simulink model "przyklad_mateusz"  (R2023a)
settings: Solver=ode1  StartTime=0.0  StopTime=inf  FixedStep=0.0001  RelTol=1e-3  EnableMultiTasking=on
undefined symbols (not defined in the file): DiscIntNeverNeededParam, sigbuilder_block
libraries: stm32f4xxblockslib x8, simulink x7, stm32blockslib x6, stmutilitieslib x3, stm32f7xxblockslib x3
(part 1 of 2)
settings Model: STM32="{\"PWMOutput\":[{\"ID\":\"stm:582\"},{\"ID\":\"stm:3\"},{\"ID\":\"stm0x2810x29OLD:3\"},{\"ID\":\"stm0x2810x29OLD:582\"}],\"DigitalPortRead\":[{\"ID\":\"stm:1051\"},{\"ID\":\"stm:7\"},{\"ID\":\"stm:347\"},{\"ID\":\"stm0x2810x29:7\"},{\"ID\":\"stm0x2810x29OLD:1051\"},{\"ID\":\"stm0x2810x29OLD:7\"},{\"ID\":\"stm0x2810x29OLD:347\"}],\"DigitalPortWrite\":[{\"ID\":\"stm:1084\"},{\"ID\":\"stm:1\"},{\"ID\":\"stm:2\"},{\"ID\":\"stm:2305\"},{\"ID\":\"stm0x2810x29:2305\"},{\"ID\":\"stm0x2810x29OLD:2305\"},{\"ID\":\"stm0x2810x29OLD:1084\"},{\"ID\":\"stm0x2810x29OLD:1\"},{\"ID\":\"stm0x2810x29OLD:2\"}],\"EncoderBlock\":[{\"ID\":\"stm:382\"},{\"ID\":\"stm:667\"},{\"ID\":\"stm:421\"},{\"ID\":\"stm0x2810x29:667\"},{\"ID\":\"stm0x2810x29:421\"},{\"ID\":\"stm0x2810x29OLD:667\"},{\"ID\":\"stm0x2810x29OLD:421\"}],\"UARTWrite\":[{\"ID\":\"stm:1060\"},{\"ID\":\"stm:1095\"},{\"ID\":\"stm:1585\"},{\"ID\":\"stm0x2810x29:1095\"},{\"ID\":\"stm0x2810x29:1060\"},{\"ID\":\"stm0x2810x29OLD:1095\"},{\"ID\":\"stm0x2810x29OLD:1060\"},{\"ID\":\"stm0x2810x29OLD:1585\"}],\"UARTRead\":[{\"ID\":\"stm:1073\"},{\"ID\":\"stm0x2810x29OLD:1073\"}],\"HardwareInterrupt\":[{\"ID\":\"stm:216\"},{\"ID\":\"stm0x2810x29OLD:216\"}],\"AnalogInput\":[{\"ID\":\"stm:2303\"},{\"ID\":\"stm0x2810x29:2303\"},{\"ID\":\"stm0x2810x29OLD:2303\"}]}"  Creator=Susze  LastModifiedBy=matim
settings SolverCC: AutoInsertRateTranBlk=on
settings OptimizationCC: EnhancedBackFolding=on  PassReuseOutputArgsAs=Individual arguments  ZeroExternalMemoryAtStartup=off  ZeroInternalMemoryAtStartup=off  MaxStackSize=64  OptimizeBlockOrder=speed  DifferentSizesBufferReuse=on  OptimizationCustomize=off  EfficientTunableParamExpr=on
settings DebuggingCC: ParameterTunabilityLossMsg=error
settings HardwareCC: ProdBitPerPointer=32  ProdBitPerSizeT=32  ProdBitPerPtrDiffT=32  ProdLargestAtomicInteger=Long  ProdLargestAtomicFloat=Double  ProdWordSize=32  ProdLongLongMode=on  ProdHWDeviceType=ARM Compatible->ARM Cortex-M
settings SFSimCC: MATLABDynamicMemAlloc=off
settings RTWCC: Description=Embedded Coder  SystemTargetFile=ert.tlc  HardwareBoard=STM32F7xx Based (Double precision FPU)  TemplateMakefile=ert_default_tmf  Toolchain=GNU Tools for ARM Embedded Processors  GPUComputeCapability=5.0
settings CodeAppCC: ForceParamTrailComments=on  IgnoreCustomStorageClasses=off  OperatorAnnotations=on  SimulinkDataObjDesc=on  SFDataObjDesc=on  InsertBlockDesc=on
settings ERTTargetCC: TargetLangStandard=C99 (ISO)  CodeReplacementLibrary=ARM Cortex-M  SupportContinuousTime=on  SupportNonInlinedSFcns=on  ExtModeTransport=3  ExtModeStaticAlloc=on  ExtModeStaticAllocSize=2048  ExtModeMexFile=ext_xcp  ExtModeIntrfLevel=Level2 - Open

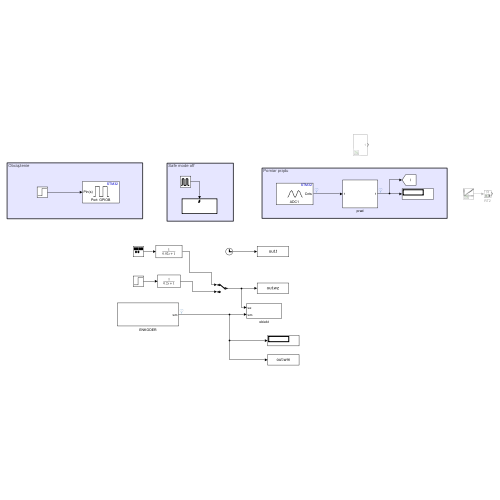
[thumbnail: Simulink's stored preview of the top-level diagram]
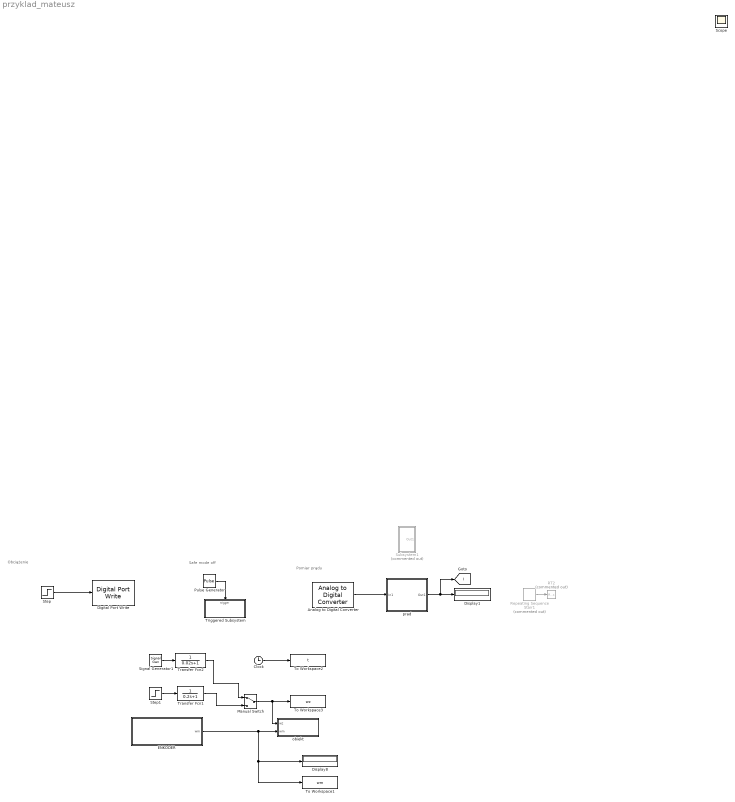
== system przyklad_mateusz ==
  note: Pomiar prądu
  note: Safe mode off
  note: Obciążenie
  Analog to Digital Converter : stm32f4xxblockslib/Analog to Digital Converter  ADCModule=ADC1  ConversionGroup=Regular  TriggerMode=Trigger and read  NumberOfConversions=1  EnableBufferConv=off  BufferLength=1  OutputStatus=off  SampleTime=-1  EnableSimPort=off  hoistedMaskSrc=ECSoC/ECSimCodegen/Analog to Digital Converter
      settings: LibrarySourceBlock=stm32f7xxblockslib/Analog to Digital Converter
  Clock : Clock
  Digital Port Write : stm32f4xxblockslib/Digital Port Write  PortName=GPIOB  PinNumber=[11]  ReadOperation=off  IOAsArray=on  EnableSimPort=off  hoistedMaskSrc=ECSoC/ECSimCodegen/Digital Port Write
      settings: LibrarySourceBlock=stm32f7xxblockslib/Digital Port Write
  Display1 : Display
  Display8 : Display
  ENKODER : Subsystem
  Manual Switch : ManualSwitch
  Pulse Generator : DiscretePulseGenerator  PulseType=Time based  Period=0.01  PulseWidth=10
  RT2 : RateTransition  Commented=on  OutPortSampleTime=0.0001
  Repeating Sequence Stair1 : simulink/Sources/Repeating Sequence Stair  Commented=on  OutValues=[0:0.1:1]  tsamp=5  OutMin=[]  OutMax=[]  OutDataTypeStr=double  OutputDataTypeScalingMode=double  OutDataType=fixdt(0,8)  ConRadixGroup=Best Precision: Vector-wise  OutScaling=2^-12
  Signal Generator1 : SignalGenerator  WaveForm=square  Amplitude=0  Frequency=0.5  Units=rad/sec
  Step : Step  Time=10  SampleTime=0
  Step1 : Step  After=0  SampleTime=0
  Subsystem1 : Subsystem  Commented=on
  To Workspace1 : ToWorkspace  VariableName=wm  SampleTime=-1
  To Workspace2 : ToWorkspace  VariableName=t  SampleTime=-1
  To Workspace3 : ToWorkspace  VariableName=wz  SampleTime=-1
  Transfer Fcn1 : TransferFcn  Denominator=[0.2 1]
  Transfer Fcn2 : TransferFcn  Denominator=[0.02 1]
  Triggered Subsystem : Subsystem  TreatAsAtomicUnit=on
  obiekt : Subsystem
  prad : Subsystem
  Scope : Scope
  tag scope: I=global
  wires:
  Pulse Generator/1 -> Triggered Subsystem/Trigger
  ENKODER/1(wm) -> Display8/1, To Workspace1/1, obiekt/2(wm)
  Clock/1 -> To Workspace2/1
  Manual Switch/1 -> obiekt/1(wz), To Workspace3/1
  Signal Generator1/1 -> Transfer Fcn2/1
  Transfer Fcn2/1 -> Manual Switch/1
  Step1/1 -> Transfer Fcn1/1
  Transfer Fcn1/1 -> Manual Switch/2
  Repeating Sequence Stair1/1 -> RT2/1
  Analog to Digital Converter/1 -> prad/1(In1)
  prad/1(Out1) -> [I], Display1/1
  Step/1 -> Digital Port Write/1

== system przyklad_mateusz/ENKODER ==
  Constant : Constant  Value=65536
  Constant1 : Constant  Value=1250
  Detect Rise Positive : simulink/Logic and Bit Operations/Detect Rise Positive  vinit=0  OutDataTypeStr=boolean
  Divide : Product  Inputs=*/
  Encoder1 : stm32blockslib/Encoder  TimerModule=TIM4  EnableResetInput=on  OutputDirection=on  SampleTime=-1
      settings: LibrarySourceBlock=stm32f7xxblockslib/Encoder
  Minus : Sum  Inputs=+-
  Pulse Generator : DiscretePulseGenerator  PulseType=Time based  Period=0.01  PulseWidth=10
  Switch : Switch  Criteria=u2 > Threshold  SaturateOnIntegerOverflow=off  InputSameDT=off
  Triggered Subsystem : Subsystem  TreatAsAtomicUnit=on
  Unit Delay : UnitDelay  SampleTime=-1  HasFrameUpgradeWarning=on
  wm : Outport
  wires:
  Detect Rise Positive/1 -> Unit Delay/1
  Switch/1 -> Triggered Subsystem/1(In1)
  Encoder1/2 -> Switch/2
  Encoder1/1 -> Switch/3, Minus/1
  Constant/1 -> Minus/2
  Minus/1 -> Switch/1
  Constant1/1 -> Divide/2
  Triggered Subsystem/1(wm) -> Divide/1
  Pulse Generator/1 -> Detect Rise Positive/1, Triggered Subsystem/Trigger
  Unit Delay/1 -> Encoder1/1
  Divide/1 -> wm/1

== system przyklad_mateusz/Subsystem1 ==
  Byte Pack1 : stmutilitieslib/Byte Pack  Commented=on  datatypes={'uint8';'uint8';'uint8';'uint8';'uint8'}  byteAlign=1  blockPlatform=stm32f4discovery
  Constant5 : Constant  Commented=on  Value=170  OutDataTypeStr=uint8
  Constant6 : Constant  Commented=on  Value=12  OutDataTypeStr=uint8
  Constant7 : Constant  Commented=on  Value=5  OutDataTypeStr=uint8
  Constant8 : Constant  Commented=on  Value=0  OutDataTypeStr=uint8
  Constant9 : Constant  Commented=on  Value=0  OutDataTypeStr=uint8
  RT : RateTransition  Commented=on  OutPortSampleTime=0.0001
  Repeating Sequence Stair : simulink/Sources/Repeating Sequence Stair  Commented=on  OutValues=[0:0.1:1]  tsamp=5  OutMin=[]  OutMax=[]  OutDataTypeStr=double  OutputDataTypeScalingMode=double  OutDataType=fixdt(0,8)  ConRadixGroup=Best Precision: Vector-wise  OutScaling=2^-12
  Signal Builder2 : Subsystem  Tag=STV Subsys  Commented=on  LoadFcn=sigbuilder_block('load');  StartFcn=sigbuilder_block('start');  StopFcn=sigbuilder_block('stop');  ClipboardFcn=sigbuilder_block('clipboard');  mask(Sigbuilder block){tuvar=[0:10]}
      mask help: Simulink:masks:SigbuilderBlock_MD
      mask init:
      | if ~strcmp(get_param(bdroot(gcbh),'SimulationStatus'),'stopped') tuvar = sigbuilder_block('maskInit'); end
      settings: CopyFcn=sigbuilder_block('copy');  DeleteFcn=sigbuilder_block('delete');  ModelCloseFcn=sigbuilder_block('modelClose');  PreSaveFcn=sigbuilder_block('preSave');  PauseFcn=sigbuilder_block('pause');  ContinueFcn=sigbuilder_block('continue');  NameChangeFcn=sigbuilder_block('namechange');  OpenFcn=sigbuilder_block('open',[5.4 36 1141.2 516.6 ]);  CloseFcn=sigbuilder_block('close');
      mask Display: plot(0, 0, 100, 100,[2, 2, 32, 32, 2], [68, 8, 8, 68, 68],[32, 2], [38, 38], [32, 19, 2],[53, 60, 44], [32, 17, 17, 2],[16, 16, 31, 31]);txt = getActiveGroup(gcbh);text(2, 100, txt,'verticalAlignment', 'top');
  Step3 : Step  Commented=on  Time=0.01  SampleTime=0
  Subsystem : Subsystem  Commented=on
  UART/USART Write1 : stm32blockslib/UART//USART Write  Commented=on  UARTModule=UART4  LengthOfDataToSend=off  BlockingMode=off  BlockingTimeout=0.1  OutputStatus=off
      settings: LibrarySourceBlock=stm32f7xxblockslib/UART//USART Write
  Out1 : Outport
  wires:
  Constant8/1 -> Byte Pack1/4
  RT/1 -> Out1/1
  Constant9/1 -> Byte Pack1/5  "prędkość 0-100"
  Constant5/1 -> Byte Pack1/1
  Constant6/1 -> Byte Pack1/2
  Byte Pack1/1 -> UART/USART Write1/1
  Repeating Sequence Stair/1 -> RT/1
  Constant7/1 -> Byte Pack1/3

== system przyklad_mateusz/Triggered Subsystem ==
  Trigger : TriggerPort  VariantControl=(inherit)
  Byte Pack1 : stmutilitieslib/Byte Pack  datatypes={'uint8';'uint8';'uint8'}  byteAlign=1  blockPlatform=stm32f4discovery
  Constant7 : Constant  Value=170  OutDataTypeStr=uint8
  Constant8 : Constant  Value=12  OutDataTypeStr=uint8
  Constant9 : Constant  Value=3  OutDataTypeStr=uint8
  UART/USART Write1 : stm32blockslib/UART//USART Write  UARTModule=UART4  LengthOfDataToSend=off  BlockingMode=off  BlockingTimeout=0.1  OutputStatus=off
      settings: LibrarySourceBlock=stm32f7xxblockslib/UART//USART Write
  wires:
  Constant9/1 -> Byte Pack1/3
  Constant8/1 -> Byte Pack1/2
  Byte Pack1/1 -> UART/USART Write1/1
  Constant7/1 -> Byte Pack1/1

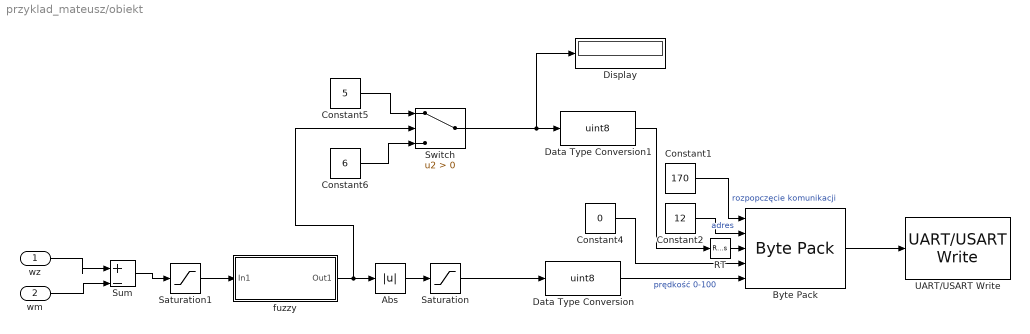
== system przyklad_mateusz/obiekt ==
  wz : Inport
  wm : Inport  Port=2
  Abs : Abs  SaturateOnIntegerOverflow=off
  Byte Pack : stmutilitieslib/Byte Pack  datatypes={'uint8';'uint8';'uint8';'uint8';'uint8'}  byteAlign=1  blockPlatform=stm32f4discovery
  Constant1 : Constant  Value=170  OutDataTypeStr=uint8
  Constant2 : Constant  Value=12  OutDataTypeStr=uint8
  Constant4 : Constant  Value=0  OutDataTypeStr=uint8
  Constant5 : Constant  Value=5  OutDataTypeStr=uint8
  Constant6 : Constant  Value=6  OutDataTypeStr=uint8
  Data Type Conversion : DataTypeConversion  OutDataTypeStr=uint8  SaturateOnIntegerOverflow=off  RndMeth=Floor
  Data Type Conversion1 : DataTypeConversion  OutDataTypeStr=uint8  SaturateOnIntegerOverflow=off  RndMeth=Floor
  Display : Display
  RT : RateTransition  OutPortSampleTime=0.0001
  Saturation : Saturate  UpperLimit=100  LowerLimit=0
  Saturation1 : Saturate  UpperLimit=1  LowerLimit=-1
  Sum : Sum  Inputs=|+-
  Switch : Switch  Criteria=u2 > Threshold  SaturateOnIntegerOverflow=off  InputSameDT=off
  UART/USART Write : stm32blockslib/UART//USART Write  UARTModule=UART4  LengthOfDataToSend=off  BlockingMode=off  BlockingTimeout=0.1  OutputStatus=off
      settings: LibrarySourceBlock=stm32f7xxblockslib/UART//USART Write
  fuzzy : Subsystem
  wires:
  Sum/1 -> Saturation1/1
  wz/1 -> Sum/1
  wm/1 -> Sum/2
  Constant2/1 -> Byte Pack/2  "adres"
  Constant1/1 -> Byte Pack/1  "rozpopczęcie komunikacji"
  Byte Pack/1 -> UART/USART Write/1
  Constant4/1 -> Byte Pack/4
  Data Type Conversion/1 -> Byte Pack/5  "prędkość 0-100"
  Constant5/1 -> Switch/1
  Constant6/1 -> Switch/3
  Switch/1 -> Data Type Conversion1/1, Display/1
  Data Type Conversion1/1 -> RT/1
  RT/1 -> Byte Pack/3
  Abs/1 -> Saturation/1
  Saturation1/1 -> fuzzy/1(In1)
  fuzzy/1(Out1) -> Abs/1, Switch/2
  Saturation/1 -> Data Type Conversion/1

== system przyklad_mateusz/prad ==
  In1 : Inport
  Constant : Constant  Value=1.65
  Gain : Gain  Gain=0.00080586
  Gain1 : Gain  Gain=15.15
  Sum : Sum  Inputs=|+-
  Transfer Fcn3 : TransferFcn  Denominator=[0.2 1]
  Out1 : Outport
  wires:
  In1/1 -> Gain/1
  Gain/1 -> Sum/1
  Constant/1 -> Sum/2
  Sum/1 -> Gain1/1
  Gain1/1 -> Transfer Fcn3/1
  Transfer Fcn3/1 -> Out1/1

== system przyklad_mateusz/ENKODER/Triggered Subsystem ==
  In1 : Inport
  Trigger : TriggerPort  VariantControl=(inherit)
  Gain : Gain  Gain=3
  wm : Outport
  wires:
  In1/1 -> Gain/1
  Gain/1 -> wm/1

== system przyklad_mateusz/Subsystem1/Signal Builder2 ==
  Demux : Demux  Tag=STV Demux  Outputs=1
      settings: DisplayOption=none
  FromWs : FromWorkspace  Tag=STV FromWs  VariableName=tuvar
      SigBuilderData=|
      | common.afterFinalStr = 'Extrapolate'
      | common.sampleTime = 0
      | dataSet.timeRange = [0 60]
      | dataSet.name = 'Group 1'
      | sbobj.Groups.Name = 'Group 1'
      | sbobj.Groups.Signals.Name = 'Prędkość'
      | sbobj.Groups.Signals.XData = [0 2 2 8 8 14 14 20 20 26 26 32 32 38 38 55.75 55.75 60]
      | sbobj.Groups.Signals.YData = [0 0 0.4 0.4 -0.395 -0.395 0.405 0.405 -0.4 -0.4 0.4 0.4 -0.4 -0.4 0.4 0.4 0 0]
      | sbobj.Groups.TimeRange = [0 60]
  Prędkość : Outport  Tag=STV Outport
  wires:
  Demux/1 -> Prędkość/1
  FromWs/1 -> Demux/1

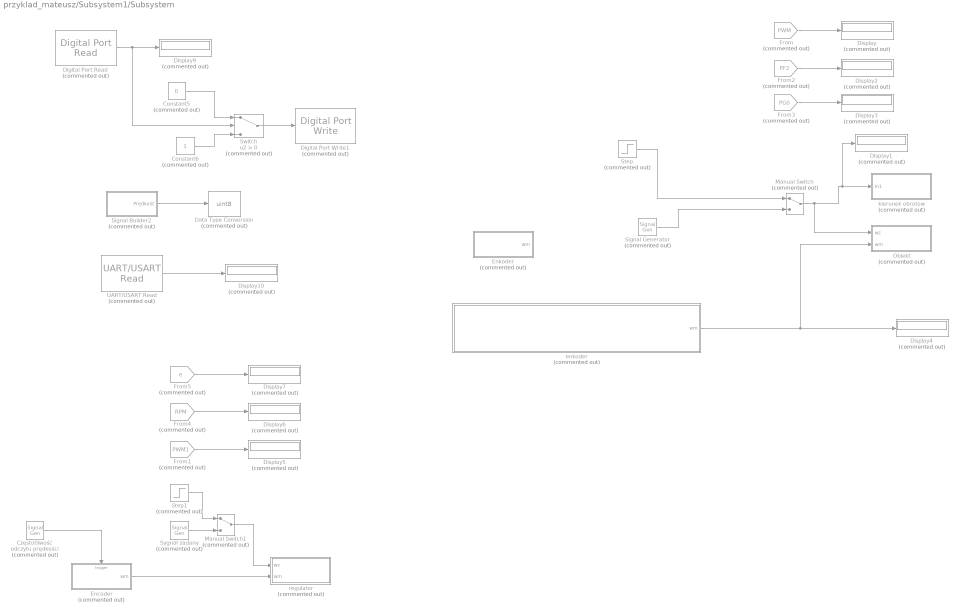
== system przyklad_mateusz/Subsystem1/Subsystem ==
  Constant5 : Constant  Commented=on  Value=0
  Constant6 : Constant  Commented=on
  Częstotliwość odczytu prędkości : SignalGenerator  Commented=on  WaveForm=square  Frequency=100
  Data Type Conversion : DataTypeConversion  Commented=on  OutDataTypeStr=uint8  SaturateOnIntegerOverflow=off  RndMeth=Floor
  Digital Port Read : stm32f4xxblockslib/Digital Port Read  Commented=on  PortName=GPIOB  PinNumber=[9]  ReadOperation=on  IOAsArray=on  SampleTime=-1  EnableSimPort=off  hoistedMaskSrc=ECSoC/ECSimCodegen/Digital Port Read
      settings: LibrarySourceBlock=stm32f7xxblockslib/Digital Port Read
  Digital Port Write1 : stm32f4xxblockslib/Digital Port Write  Commented=on  PortName=GPIOB  PinNumber=[8]  ReadOperation=off  IOAsArray=on  EnableSimPort=off  hoistedMaskSrc=ECSoC/ECSimCodegen/Digital Port Write
      settings: LibrarySourceBlock=stm32f7xxblockslib/Digital Port Write
  Display{,1..7,9..10} (10 alike) : Display  Commented=on
  Encoder : Subsystem  Commented=on  TreatAsAtomicUnit=on
  Enkoder : Subsystem  Commented=on
  From : From  Commented=on  GotoTag=PWM  TagVisibility=global
  From1 : From  Commented=on  GotoTag=PWM1
  From2 : From  Commented=on  GotoTag=PF2  TagVisibility=global
  From3 : From  Commented=on  GotoTag=PG0  TagVisibility=global
  From4 : From  Commented=on  GotoTag=RPM  TagVisibility=global
  From5 : From  Commented=on  GotoTag=e
  Manual Switch : ManualSwitch  Commented=on
  Manual Switch1 : ManualSwitch  Commented=on
  Obiekt : Subsystem  Commented=on
  Signal Generator : SignalGenerator  Commented=on  WaveForm=square  Frequency=0.1  Units=rad/sec
  Signal Builder2 : Subsystem  Tag=STV Subsys  Commented=on  LoadFcn=sigbuilder_block('load');  StartFcn=sigbuilder_block('start');  StopFcn=sigbuilder_block('stop');  ClipboardFcn=sigbuilder_block('clipboard');  mask(Sigbuilder block){tuvar=[0:10]}
      mask help: Simulink:masks:SigbuilderBlock_MD
      mask init:
      | if ~strcmp(get_param(bdroot(gcbh),'SimulationStatus'),'stopped') tuvar = sigbuilder_block('maskInit'); end
      settings: CopyFcn=sigbuilder_block('copy');  DeleteFcn=sigbuilder_block('delete');  ModelCloseFcn=sigbuilder_block('modelClose');  PreSaveFcn=sigbuilder_block('preSave');  PauseFcn=sigbuilder_block('pause');  ContinueFcn=sigbuilder_block('continue');  NameChangeFcn=sigbuilder_block('namechange');  OpenFcn=sigbuilder_block('open',[0 36 1152 555.6 ]);  CloseFcn=sigbuilder_block('close');
      mask Display: plot(0, 0, 100, 100,[2, 2, 32, 32, 2], [68, 8, 8, 68, 68],[32, 2], [38, 38], [32, 19, 2],[53, 60, 44], [32, 17, 17, 2],[16, 16, 31, 31]);txt = getActiveGroup(gcbh);text(2, 100, txt,'verticalAlignment', 'top');
  Step : Step  Commented=on  SampleTime=0
  Step1 : Step  Commented=on  After=200  SampleTime=0
  Switch : Switch  Commented=on  Criteria=u2 > Threshold  SaturateOnIntegerOverflow=off  InputSameDT=off
  Sygnał zadany : SignalGenerator  Commented=on  WaveForm=square  Amplitude=0.5  Frequency=0.1
  UART/USART Read : stm32blockslib/UART//USART Read  Commented=on  UARTModule=UART4  DataType=uint8  DataLength=1  BlockingMode=off  BlockingTimeout=0.1  OutputLength=off  OutputStatus=off  SampleTime=-1
      settings: LibrarySourceBlock=stm32f7xxblockslib/UART//USART Read
  enkoder : Subsystem  Commented=on
  kierunek obrotow : Subsystem  Commented=on
  regulator : Subsystem  Commented=on
  wires:
  Digital Port Read/1 -> Switch/2, Display9/1
  Switch/1 -> Digital Port Write1/1
  Constant5/1 -> Switch/1
  Signal Builder2/1(Prędkość) -> Data Type Conversion/1
  Constant6/1 -> Switch/3
  UART/USART Read/1 -> Display10/1
  Step1/1 -> Manual Switch1/1
  From5/1 -> Display7/1
  Częstotliwość odczytu prędkości/1 -> Encoder/Trigger
  Sygnał zadany/1 -> Manual Switch1/2
  Manual Switch1/1 -> regulator/1(wz)
  From1/1 -> Display5/1
  Encoder/1(wm) -> regulator/2(wm)
  From4/1 -> Display6/1
  From2/1 -> Display2/1
  From3/1 -> Display3/1
  enkoder/1(wm) -> Obiekt/2(wm), Display4/1
  Step/1 -> Manual Switch/1
  Signal Generator/1 -> Manual Switch/2
  Manual Switch/1 -> Obiekt/1(wz), Display1/1, kierunek obrotow/1(In1)
  From/1 -> Display/1

== system przyklad_mateusz/obiekt/fuzzy ==
  In1 : Inport
  Discrete Derivative : simulink/Discrete/Discrete Derivative  gainval=1.0  ICPrevScaledInput=0.0  OutMin=[]  OutMax=[]  OutDataType=fixdt(1, 16)  OutScaling=2^-10  DoSatur=off
  Discrete-Time Integrator : DiscreteIntegrator  SampleTime=-1  ICPrevOutput=DiscIntNeverNeededParam  ICPrevScaledInput=DiscIntNeverNeededParam
  Fuzzy Logic Controller : Subsystem  Commented=on
      mask help: Simulink:masks:GenSFuncDesc_MD
      mask Help: eval('feval(''rtwprivate'',''rtwhelpview'',''rtw_sfcn_block'')');
      mask Display:
      | iconStr = fuzzy.internal.utility.getMaskDisplayString;
      | eval(iconStr)
  Fuzzy Type 1 : Subsystem  Commented=on
  Fuzzy Type 2 : Subsystem
  Gain : Gain  Gain=2
  Gain1 : Gain  Gain=0.05
  Gain2 : Gain  Gain=300
  Mux : Mux  Commented=on  Inputs=2
  Saturation : Saturate  UpperLimit=1  LowerLimit=-1
  Saturation1 : Saturate  UpperLimit=1  LowerLimit=-1
  Out1 : Outport
  wires:
  In1/1 -> Discrete Derivative/1, Gain/1
  Gain/1 -> Saturation/1
  Discrete Derivative/1 -> Gain1/1
  Gain1/1 -> Saturation1/1
  Gain2/1 -> Discrete-Time Integrator/1
  Discrete-Time Integrator/1 -> Out1/1
  Mux/1 -> Fuzzy Logic Controller/1(in)
  Saturation1/1 -> Fuzzy Type 2/2(de1)
  Saturation/1 -> Fuzzy Type 2/1(e2)
  Fuzzy Type 2/1(du) -> Gain2/1

== system przyklad_mateusz/Subsystem1/Subsystem/Encoder ==
  Trigger : TriggerPort  TriggerType=falling  VariantControl=(inherit)
  Add : Sum
  Constant3 : Constant  Value=65536
  Display : Display
  Encoder : stm32blockslib/Encoder  TimerModule=TIM4  EnableResetInput=on  OutputDirection=on  SampleTime=-1
      settings: LibrarySourceBlock=stm32f7xxblockslib/Encoder
  Gain : Gain  Gain=6
  Subtract : Sum  Inputs=+-
  Subtract1 : Sum  Inputs=+-
  Switch : Switch  Criteria=u2 > Threshold  SaturateOnIntegerOverflow=off  InputSameDT=off
  Unit Delay : UnitDelay  SampleTime=-1  HasFrameUpgradeWarning=on
  wm : Outport
  tag scope: RPM=global
  wires:
  Subtract/1 -> Switch/2, Switch/1
  Switch/1 -> Gain/1
  Add/1 -> Switch/3
  Constant3/1 -> Subtract1/1
  Subtract1/1 -> Add/2
  Encoder/1 -> Unit Delay/1, Add/1, Subtract/1
  Unit Delay/1 -> Subtract1/2, Subtract/2
  Gain/1 -> [RPM], wm/1
  Encoder/2 -> Display/1

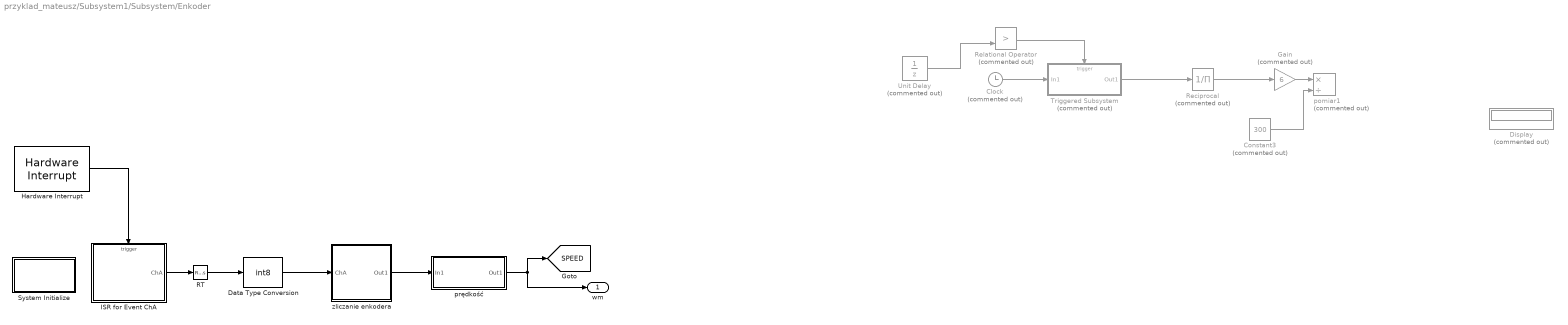
== system przyklad_mateusz/Subsystem1/Subsystem/Enkoder ==
  Clock : Clock  Commented=on
  Constant3 : Constant  Commented=on  Value=300
  Data Type Conversion : DataTypeConversion  OutDataTypeStr=int8  SaturateOnIntegerOverflow=off  RndMeth=Floor
  Display : Display  Commented=on
  Gain : Gain  Commented=on  Gain=6
  Hardware Interrupt : stm32f7xxblockslib/Hardware Interrupt  ISRGroup=External interrupts (EXTI)  ISRName=EXTI3_IRQHandler  ISRNumber=24  EventsList={ 'on', 'EXTI3 Event', '1'; 'off', 'Custom event', '2' }  SelectedEvents={'EXTI3 Event'}  TaskPriority=30  DisablePreemption=off  ClearInterruptFlagsAtEndOfEvent=off  InterruptDefinitionFile=$(TARGET_ROOT)/registry/interrupts/STM32F4xxBased_interrupts.xml  HardwareBoard=STM32F7xx Based  EnableSimPort=off
  ISR for Event ChA : Subsystem  TreatAsAtomicUnit=on
  RT : RateTransition  Deterministic=off  OutPortSampleTime=0.001
  Reciprocal : Product  Commented=on  Inputs=/
  Relational Operator : RelationalOperator  Commented=on  Operator=>  OutDataTypeStr=boolean  RndMeth=Simplest  InputSameDT=off
  System Initialize : Subsystem  mask(System Initialize){ShowInLibBrowser=0}
      mask prompts: ShowInLibBrowser "Simulink:masks:CustCodeMaskParam1_MP"
      settings: CopyFcn=cccopyfcn(gcb)  OpenFcn=ccopenfcn('System Initialize Function')
      mask Help: eval('feval(''rtwprivate'',''rtwhelpview'',''rtw_sys_initialize_block'')');
      mask Display: disp('System\nInitialize');
  Triggered Subsystem : Subsystem  Commented=on  TreatAsAtomicUnit=on
  Unit Delay : UnitDelay  Commented=on  SampleTime=-1  HasFrameUpgradeWarning=on
  pomiar1 : Product  Commented=on  Inputs=*/
  prędkość : Subsystem
  zliczanie enkodera : Subsystem
  wm : Outport
  tag scope: SPEED=global
  wires:
  Hardware Interrupt/1 -> ISR for Event ChA/Trigger
  Triggered Subsystem/1(Out1) -> Reciprocal/1
  Relational Operator/1 -> Triggered Subsystem/Trigger
  Clock/1 -> Triggered Subsystem/1(In1)
  Constant3/1 -> pomiar1/2
  Reciprocal/1 -> Gain/1
  Gain/1 -> pomiar1/1
  ? -> Relational Operator/1, Unit Delay/1
  Unit Delay/1 -> Relational Operator/2
  RT/1 -> Data Type Conversion/1
  Data Type Conversion/1 -> zliczanie enkodera/1(ChA)
  zliczanie enkodera/1(Out1) -> prędkość/1(In1)
  prędkość/1(Out1) -> wm/1, [SPEED]
  ISR for Event ChA/1(ChA) -> RT/1

== system przyklad_mateusz/Subsystem1/Subsystem/Obiekt ==
  wz : Inport
  wm : Inport  Port=2
  Constant : Constant  Value=80
  Manual Switch : ManualSwitch  CurrentSetting=0
  Moj : Subsystem
  PWM Output : stm32f7xxblockslib/PWM Output  TimerModule=TIM1  DutycycleUnits=Percentage  EnableChannel1=on  EnableChannel2=off  EnableChannel3=off  EnableChannel4=off  EnableChannel5=off  EnableChannel6=off  EnableCounterInput=off  EnableMainOutputInput=off  EnableFrequencyInput=off  SetRCAfterCE=off  OutputDirection=off  OutputMainOutputEnableStatus=off  SampleTime=0.1  EnableSimPort=off  EnableUpdateEvent=off  EnableCaptureCompare1Event=off  EnableCaptureCompare2Event=off  EnableCaptureCompare3Event=off  EnableCaptureCompare4Event=off  EnableTriggerEvent=off  EnableBreakEvent=off  EnableBreakEvent2=off  ProcessorFamily=STM32F7  hoistedMaskSrc=ECSoC/ECSimCodegen/PWM Output
  Saturation : Saturate  UpperLimit=100  LowerLimit=0
  Sum : Sum  Inputs=|+-
  tag scope: PWM=global
  wires:
  Sum/1 -> Moj/1(In1)
  Moj/1(Out1) -> Saturation/1
  wz/1 -> Sum/1
  wm/1 -> Sum/2
  Saturation/1 -> Manual Switch/2
  Constant/1 -> Manual Switch/1
  Manual Switch/1 -> [PWM], PWM Output/1

== system przyklad_mateusz/Subsystem1/Subsystem/Signal Builder2 ==
  Demux : Demux  Tag=STV Demux  Outputs=1
      settings: DisplayOption=none
  FromWs : FromWorkspace  Tag=STV FromWs  VariableName=tuvar
      SigBuilderData=|
      | common.afterFinalStr = 'Extrapolate'
      | common.sampleTime = 0
      | dataSet.timeRange = [0 40]
      | dataSet.name = 'Group 1'
      | sbobj.Groups.Name = 'Group 1'
      | sbobj.Groups.Signals.Name = 'Prędkość'
      | sbobj.Groups.Signals.XData = [0 5 5 10 10 15 15 20 20 25 25 30 30 35 35 40]
      | sbobj.Groups.Signals.YData = [0 0 20 20 30 30 40 40 50 50 60 60 70 70 80.2 80.2]
      | sbobj.Groups.TimeRange = [0 40]
  Prędkość : Outport  Tag=STV Outport
  wires:
  Demux/1 -> Prędkość/1
  FromWs/1 -> Demux/1

== system przyklad_mateusz/Subsystem1/Subsystem/enkoder ==
  Clock : Clock
  Constant3 : Constant  Value=300
  Data Type Conversion : DataTypeConversion  OutDataTypeStr=uint8  SaturateOnIntegerOverflow=off  RndMeth=Floor
  Digital Port Read : stm32f4xxblockslib/Digital Port Read  PortName=GPIOA  PinNumber=[3]  ReadOperation=on  IOAsArray=on  SampleTime=-1  EnableSimPort=off  hoistedMaskSrc=ECSoC/ECSimCodegen/Digital Port Read
      settings: LibrarySourceBlock=stm32f7xxblockslib/Digital Port Read
  Gain : Gain  Gain=6
  Reciprocal : Product  Inputs=/
  Relational Operator : RelationalOperator  Operator=>  OutDataTypeStr=boolean  RndMeth=Simplest  InputSameDT=off
  Triggered Subsystem : Subsystem  TreatAsAtomicUnit=on
  Unit Delay : UnitDelay  SampleTime=-1  HasFrameUpgradeWarning=on
  pomiar1 : Product  Inputs=*/
  wm : Outport
  wires:
  Digital Port Read/1 -> Relational Operator/1, Unit Delay/1
  Clock/1 -> Triggered Subsystem/1(In1)
  Triggered Subsystem/1(Out1) -> Reciprocal/1
  Unit Delay/1 -> Relational Operator/2
  Gain/1 -> pomiar1/1
  Reciprocal/1 -> Gain/1
  Constant3/1 -> pomiar1/2
  Relational Operator/1 -> Triggered Subsystem/Trigger
  pomiar1/1 -> wm/1

== system przyklad_mateusz/Subsystem1/Subsystem/kierunek obrotow ==
  In1 : Inport
  Digital Port Write : stm32f4xxblockslib/Digital Port Write  PortName=GPIOG  PinNumber=[0]  ReadOperation=off  IOAsArray=on  EnableSimPort=off  hoistedMaskSrc=ECSoC/ECSimCodegen/Digital Port Write
      settings: LibrarySourceBlock=stm32f7xxblockslib/Digital Port Write
  Digital Port Write1 : stm32f4xxblockslib/Digital Port Write  PortName=GPIOF  PinNumber=[2]  ReadOperation=off  IOAsArray=on  EnableSimPort=off  hoistedMaskSrc=ECSoC/ECSimCodegen/Digital Port Write
      settings: LibrarySourceBlock=stm32f7xxblockslib/Digital Port Write
  kierunek obrotów : Subsystem
  tag scope: PF2=global, PG0=global
  wires:
  In1/1 -> kierunek obrotów/1(u)
  kierunek obrotów/1(y) -> Digital Port Write/1, [PG0]
  kierunek obrotów/2(Out2) -> [PF2], Digital Port Write1/1

== system przyklad_mateusz/Subsystem1/Subsystem/regulator ==
  wz : Inport
  wm : Inport  Port=2
  Constant : Constant  Value=80
  Manual Switch : ManualSwitch  CurrentSetting=0
  PWM Output : stm32f7xxblockslib/PWM Output  TimerModule=TIM1  DutycycleUnits=Percentage  EnableChannel1=on  EnableChannel2=off  EnableChannel3=off  EnableChannel4=off  EnableChannel5=off  EnableChannel6=off  EnableCounterInput=off  EnableMainOutputInput=off  EnableFrequencyInput=off  SetRCAfterCE=off  OutputDirection=off  OutputMainOutputEnableStatus=off  SampleTime=0.1  EnableSimPort=off  EnableUpdateEvent=off  EnableCaptureCompare1Event=off  EnableCaptureCompare2Event=off  EnableCaptureCompare3Event=off  EnableCaptureCompare4Event=off  EnableTriggerEvent=off  EnableBreakEvent=off  EnableBreakEvent2=off  ProcessorFamily=STM32F7  hoistedMaskSrc=ECSoC/ECSimCodegen/PWM Output
  Saturation : Saturate  UpperLimit=100  LowerLimit=0
  Sum : Sum  Inputs=|+-
  fuzzy : Subsystem
  tag scope: PWM1=global, e=global
  wires:
  Sum/1 -> [e], fuzzy/1(In1)
  fuzzy/1(Out1) -> Saturation/1
  wz/1 -> Sum/1
  wm/1 -> Sum/2
  Saturation/1 -> Manual Switch/2
  Constant/1 -> Manual Switch/1
  Manual Switch/1 -> [PWM1], PWM Output/1

== system przyklad_mateusz/obiekt/fuzzy/Fuzzy Logic Controller ==
  in : Inport
  Fuzzy Logic Controller_sfcn : S-Function  FunctionName=Fuzzy0_sf  SFunctionModules=""  SFunctionDeploymentMode=off  EnableBusSupport=off  mask{rtw_sf_name=Fuzzy0_sf, showVar=off}
      mask prompts: rtw_sf_name "Simulink:masks:GenSFuncName_MP"; showVar "Simulink:masks:GenSFuncShowModuleList_MP"
      mask help: Simulink:masks:GenSFuncDesc_MD
      mask init:
      | displist = '';
      | if ~strcmp(get_param(gcb, 'FunctionName'), rtw_sf_name);
      |   set_param(gcb, 'FunctionName', rtw_sf_name);
      | end
      | % Check if we are generating code
      | rtw_mode = false;
      | if strcmpi(get_param(bdroot(gcb),'SimulationStatus'),'Initializing')
      | 	rtw_mode = strcmpi(get_param(bdroot(gcb),'BuildingRTWCode'),'on') && ...
      | 		~strcmpi(get_param(bdroot(gcb),'TargetStyle'),'SimulationTarget');
      | end
      | if showVar || rtw_mode
      | 	if exist('rtwsfunc') == 2 | exist('rtwsfunc') == 6
      | 		tmplist = rtwsfunc(rtw_sf_name,gcb);
      | 		tmplist = DAStudio.message('Simulink:masks:GenSFuncListOfModules_IC', tmplist);
      | 	elseif showVar
      | 		tmplist1 = DAStudio.message('Simulink:masks:GenSFuncListOfModules_IC', '');
      |         tmplist2 = DAStudio.message('Simulink:masks:GenSFuncNotLicensed_IC');
      |         tmplist = [tmplist1 tmplist2];
      |  	end
      | end
      | if showVar
      |   displist = tmplist;
      | end
      settings: CopyFcn=|
      | if ~strcmp(get_param(gcb,'Linkstatus'),'none') && ...
      | ~strcmp(get_param(gcb,'Linkstatus'),'implicit')
      |   set_param(gcb,'LinkStatus','none');
      | end
      mask Help: eval('feval(''rtwprivate'',''rtwhelpview'',''rtw_sfcn_block'')');
      mask Display:
      | port_label('input',1,'in');
      | port_label('output',1,'out');
  __InputSSForSFun__ : Subsystem
  __OutputSSForSFun__ : Subsystem
  out : Outport  VectorParamsAs1DForOutWhenUnconnected=off
  wires:
  in/1 -> __InputSSForSFun__/1(in)
  __InputSSForSFun__/1(__UniqueOutportName__1__) -> Fuzzy Logic Controller_sfcn/1
  Fuzzy Logic Controller_sfcn/1 -> __OutputSSForSFun__/1(__UniqueInportName__1__)
  __OutputSSForSFun__/1(out) -> out/1

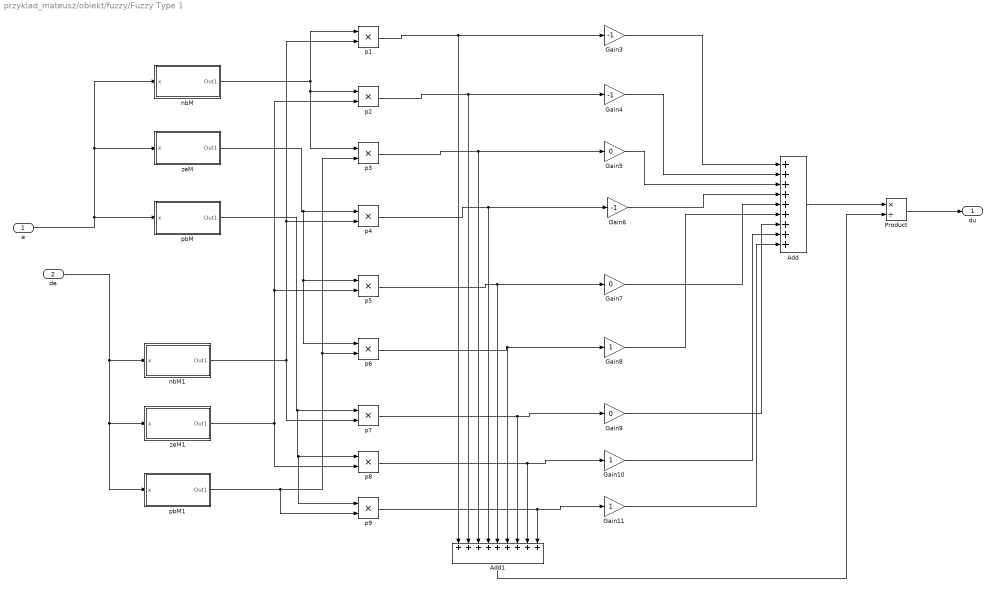
== system przyklad_mateusz/obiekt/fuzzy/Fuzzy Type 1 ==
  e : Inport
  de : Inport  Port=2
  Add : Sum  Inputs=+++++++++
  Add1 : Sum  Inputs=+++++++++
  Gain10 : Gain
  Gain11 : Gain
  Gain3 : Gain  Gain=-1
  Gain4 : Gain  Gain=-1
  Gain5 : Gain  Gain=0
  Gain6 : Gain  Gain=-1
  Gain7 : Gain  Gain=0
  Gain8 : Gain
  Gain9 : Gain  Gain=0
  Product : Product  Inputs=*/
  nbM : Subsystem
  nbM1 : Subsystem
  p{1..9} (9 alike) : Product
  pbM : Subsystem
  pbM1 : Subsystem
  zeM : Subsystem
  zeM1 : Subsystem
  du : Outport
  wires:
  p6/1 -> Gain8/1, Add1/6
  p8/1 -> Gain10/1, Add1/8
  p3/1 -> Gain5/1, Add1/3
  e/1 -> zeM/1(x), nbM/1(x), pbM/1(x)
  zeM1/1(Out1) -> p8/2, p5/2, p2/2
  nbM1/1(Out1) -> p7/2, p4/2, p1/2
  pbM/1(Out1) -> p9/1, p8/1, p7/1
  Gain9/1 -> Add/7
  p5/1 -> Gain7/1, Add1/5
  de/1 -> nbM1/1(x), zeM1/1(x), pbM1/1(x)
  Gain5/1 -> Add/3
  pbM1/1(Out1) -> p9/2, p6/2, p3/2
  Gain6/1 -> Add/4
  Gain4/1 -> Add/2
  p7/1 -> Gain9/1, Add1/7
  zeM/1(Out1) -> p6/1, p5/1, p4/1
  nbM/1(Out1) -> p3/1, p2/1, p1/1
  Gain7/1 -> Add/5
  p2/1 -> Gain4/1, Add1/2
  p4/1 -> Gain6/1, Add1/4
  Gain3/1 -> Add/1
  Gain11/1 -> Add/9
  Gain8/1 -> Add/6
  p1/1 -> Add1/1, Gain3/1
  Gain10/1 -> Add/8
  p9/1 -> Gain11/1, Add1/9
  Add1/1 -> Product/2
  Add/1 -> Product/1
  Product/1 -> du/1

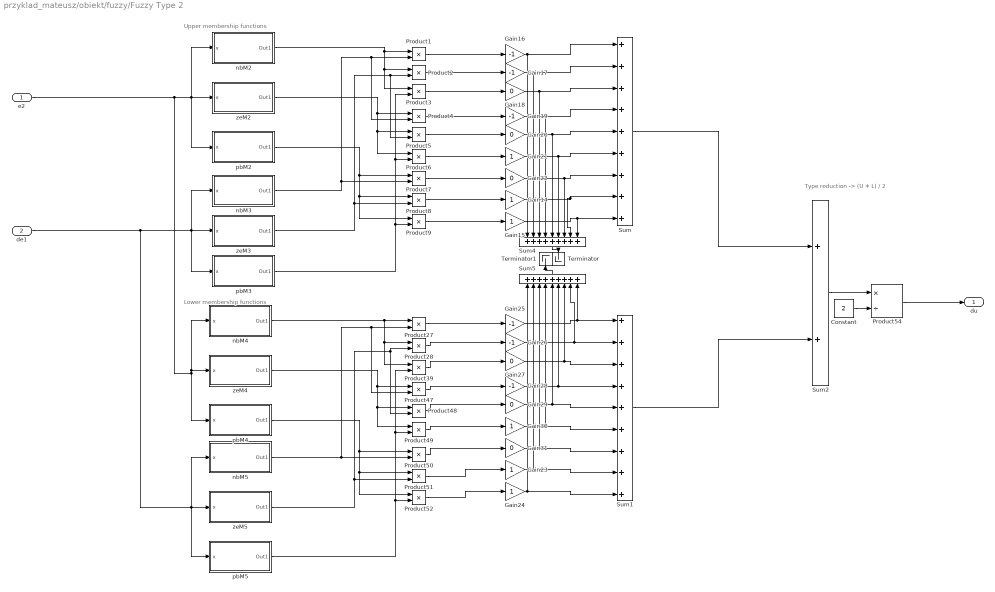
== system przyklad_mateusz/obiekt/fuzzy/Fuzzy Type 2 ==
  note: Type reduction -> (U + L) / 2
  note: Lower membership functions
  note: Upper membership functions
  e2 : Inport
  de1 : Inport  Port=2
  Constant : Constant  Value=2
  Gain{14..15,21,23..24,30} (6 alike) : Gain
  Gain{16..17,19,25..26,28} (6 alike) : Gain  Gain=-1
  Gain{18,20,22,27,29,31} (6 alike) : Gain  Gain=0
  Product{1..9,27..28,39,47..52} (18 alike) : Product
  Product54 : Product  Inputs=*/
  Sum{,1,4..5} (4 alike) : Sum  Inputs=9
  Sum2 : Sum  Inputs=2
  Terminator : Terminator
  Terminator1 : Terminator
  nbM2 : Subsystem
  nbM3 : Subsystem
  nbM4 : Subsystem
  nbM5 : Subsystem
  pbM2 : Subsystem
  pbM3 : Subsystem
  pbM4 : Subsystem
  pbM5 : Subsystem
  zeM2 : Subsystem
  zeM3 : Subsystem
  zeM4 : Subsystem
  zeM5 : Subsystem
  du : Outport
  wires:
  Product2/1 -> Gain17/1
  Sum/1 -> Sum2/1
  Product49/1 -> Gain30/1
  Product51/1 -> Gain23/1
  nbM4/1(Out1) -> Product39/1, Product28/1, Product27/1
  e2/1 -> pbM4/1(x), zeM4/1(x), nbM4/1(x), pbM2/1(x), zeM2/1(x), nbM2/1(x)
  Product52/1 -> Gain24/1
  Product27/1 -> Gain25/1
  pbM5/1(Out1) -> Product39/2, Product49/2, Product52/2
  Gain30/1 -> Sum5/4, Sum1/6
  Gain19/1 -> Sum4/4, Sum/4
  Product48/1 -> Gain29/1
  Product5/1 -> Gain20/1
  zeM5/1(Out1) -> Product28/2, Product48/2, Product51/2
  Product54/1 -> du/1
  nbM2/1(Out1) -> Product3/1, Product2/1, Product1/1
  Product39/1 -> Gain27/1
  Sum5/1 -> Terminator1/1
  Product9/1 -> Gain15/1
  Gain28/1 -> Sum5/6, Sum1/4
  Product47/1 -> Gain28/1
  Gain15/1 -> Sum4/9, Sum/9
  Gain26/1 -> Sum5/8, Sum1/2
  Sum1/1 -> Sum2/2
  Constant/1 -> Product54/2
  de1/1 -> nbM3/1(x), zeM3/1(x), pbM3/1(x), pbM5/1(x), zeM5/1(x), nbM5/1(x)
  Gain25/1 -> Sum1/1, Sum5/9
  Sum2/1 -> Product54/1
  Gain17/1 -> Sum/2, Sum4/2
  Gain23/1 -> Sum5/2, Sum1/8
  Gain27/1 -> Sum1/3, Sum5/7
  zeM4/1(Out1) -> Product47/1, Product48/1, Product49/1
  Gain31/1 -> Sum5/3, Sum1/7
  Product6/1 -> Gain21/1
  Gain18/1 -> Sum4/3, Sum/3
  Product50/1 -> Gain31/1
  Gain22/1 -> Sum4/7, Sum/7
  zeM3/1(Out1) -> Product8/2, Product5/2, Product2/2
  Product1/1 -> Gain16/1
  Product8/1 -> Gain14/1
  Gain16/1 -> Sum4/1, Sum/1
  Gain21/1 -> Sum4/6, Sum/6
  Product7/1 -> Gain22/1
  Gain20/1 -> Sum4/5, Sum/5
  nbM5/1(Out1) -> Product47/2, Product27/2, Product50/2
  Gain14/1 -> Sum4/8, Sum/8
  Product3/1 -> Gain18/1
  Gain29/1 -> Sum5/5, Sum1/5
  Product28/1 -> Gain26/1
  pbM3/1(Out1) -> Product9/2, Product6/2, Product3/2
  pbM4/1(Out1) -> Product52/1, Product51/1, Product50/1
  Gain24/1 -> Sum1/9, Sum5/1
  Product4/1 -> Gain19/1
  zeM2/1(Out1) -> Product6/1, Product5/1, Product4/1
  Sum4/1 -> Terminator/1
  nbM3/1(Out1) -> Product7/2, Product4/2, Product1/2
  pbM2/1(Out1) -> Product8/1, Product9/1, Product7/1

== system przyklad_mateusz/Subsystem1/Subsystem/Enkoder/ISR for Event ChA ==
  function : TriggerPort  TriggerType=function-call  VariantControl=(inherit)
  Digital Port Read : stm32f4xxblockslib/Digital Port Read  PortName=GPIOA  PinNumber=[3]  ReadOperation=on  IOAsArray=on  SampleTime=-1  EnableSimPort=off  hoistedMaskSrc=ECSoC/ECSimCodegen/Digital Port Read
      settings: LibrarySourceBlock=stm32f7xxblockslib/Digital Port Read
  ChA : Outport
  wires:
  Digital Port Read/1 -> ChA/1

== system przyklad_mateusz/Subsystem1/Subsystem/Enkoder/System Initialize ==

== system przyklad_mateusz/Subsystem1/Subsystem/Enkoder/Triggered Subsystem ==
  In1 : Inport
  Trigger : TriggerPort  VariantControl=(inherit)
  Subtract : Sum  Inputs=+-
  Unit Delay : UnitDelay  SampleTime=-1  HasFrameUpgradeWarning=on
  Out1 : Outport
  wires:
  In1/1 -> Subtract/1, Unit Delay/1
  Unit Delay/1 -> Subtract/2
  Subtract/1 -> Out1/1

== system przyklad_mateusz/Subsystem1/Subsystem/Enkoder/prędkość ==
  In1 : Inport
  Constant7 : Constant  Value=10  OutDataTypeStr=single
  Constant8 : Constant  Value=60  OutDataTypeStr=single
  Discrete Derivative : simulink/Discrete/Discrete Derivative  gainval=1.0  ICPrevScaledInput=0.0  OutMin=[]  OutMax=[]  OutDataType=fixdt(1, 16)  OutScaling=2^-10  DoSatur=off
  Divide1 : Product  Inputs=*/
  Product2 : Product
  Out1 : Outport
  wires:
  In1/1 -> Discrete Derivative/1
  Product2/1 -> Out1/1
  Divide1/1 -> Product2/1
  Constant7/1 -> Divide1/2
  Discrete Derivative/1 -> Divide1/1
  Constant8/1 -> Product2/2

== system przyklad_mateusz/Subsystem1/Subsystem/Enkoder/zliczanie enkodera ==
  ChA : Inport
  Add2 : Sum  Inputs=+-
  Constant : Constant  OutDataTypeStr=single
  Constant1 : Constant  OutDataTypeStr=single
  If : If  IfExpression=u1 == 1  ShowElse=off
  If Action Subsystem : Subsystem  TreatAsAtomicUnit=on
  If Action Subsystem2 : Subsystem  TreatAsAtomicUnit=on
  If1 : If  IfExpression=u1 == 0  ShowElse=off
  Memory : Memory  InheritSampleTime=on
  Out1 : Outport
  wires:
  Constant/1 -> If Action Subsystem/2(Input2)
  ChA/1 -> If1/1, If/1, Memory/1
  Constant1/1 -> If Action Subsystem2/2(Input2)
  If Action Subsystem/1(Out1) -> Add2/1
  If1/1 -> If Action Subsystem2/Action
  If Action Subsystem2/1(Out1) -> Add2/2
  If/1 -> If Action Subsystem/Action
  Add2/1 -> Out1/1
  Memory/1 -> If Action Subsystem2/1(Input), If Action Subsystem/1(Input)

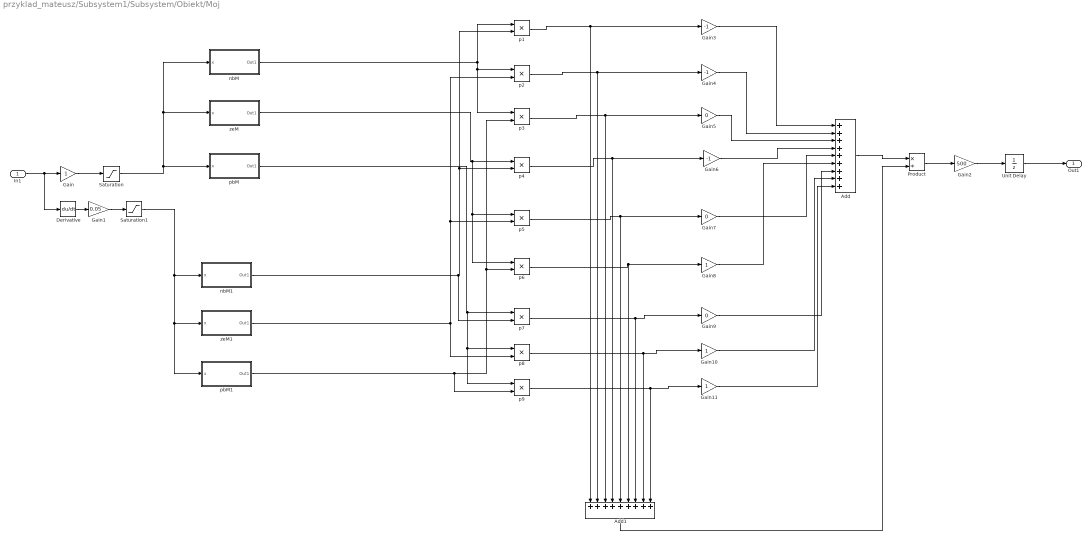
== system przyklad_mateusz/Subsystem1/Subsystem/Obiekt/Moj ==
  In1 : Inport
  Add : Sum  Inputs=+++++++++
  Add1 : Sum  Inputs=+++++++++
  Derivative : Derivative
  Gain{,8,10..11} (4 alike) : Gain
  Gain1 : Gain  Gain=0.05
  Gain2 : Gain  Gain=500
  Gain3 : Gain  Gain=-1
  Gain4 : Gain  Gain=-1
  Gain5 : Gain  Gain=0
  Gain6 : Gain  Gain=-1
  Gain7 : Gain  Gain=0
  Gain9 : Gain  Gain=0
  Product : Product  Inputs=*/
  Saturation : Saturate  UpperLimit=1  LowerLimit=-1
  Saturation1 : Saturate  UpperLimit=1  LowerLimit=-1
  Unit Delay : UnitDelay  SampleTime=-1  HasFrameUpgradeWarning=on
  nbM : Subsystem
  nbM1 : Subsystem
  p{1..9} (9 alike) : Product
  pbM : Subsystem
  pbM1 : Subsystem
  zeM : Subsystem
  zeM1 : Subsystem
  Out1 : Outport
  wires:
  In1/1 -> Derivative/1, Gain/1
  Gain/1 -> Saturation/1
  Derivative/1 -> Gain1/1
  Gain1/1 -> Saturation1/1
  Gain2/1 -> Unit Delay/1
  Product/1 -> Gain2/1
  Saturation/1 -> zeM/1(x), nbM/1(x), pbM/1(x)
  Saturation1/1 -> nbM1/1(x), zeM1/1(x), pbM1/1(x)
  p1/1 -> Add1/1, Gain3/1
  p3/1 -> Gain5/1, Add1/3
  p2/1 -> Gain4/1, Add1/2
  p4/1 -> Gain6/1, Add1/4
  p5/1 -> Gain7/1, Add1/5
  p6/1 -> Gain8/1, Add1/6
  p7/1 -> Gain9/1, Add1/7
  p8/1 -> Gain10/1, Add1/8
  p9/1 -> Gain11/1, Add1/9
  nbM/1(Out1) -> p3/1, p2/1, p1/1
  nbM1/1(Out1) -> p7/2, p4/2, p1/2
  zeM1/1(Out1) -> p8/2, p5/2, p2/2
  pbM1/1(Out1) -> p9/2, p6/2, p3/2
  zeM/1(Out1) -> p6/1, p5/1, p4/1
  pbM/1(Out1) -> p9/1, p8/1, p7/1
  Gain3/1 -> Add/1
  Gain4/1 -> Add/2
  Gain5/1 -> Add/3
  Gain6/1 -> Add/4
  Gain7/1 -> Add/5
  Gain8/1 -> Add/6
  Gain9/1 -> Add/7
  Gain10/1 -> Add/8
  Gain11/1 -> Add/9
  Add/1 -> Product/1
  Add1/1 -> Product/2
  Unit Delay/1 -> Out1/1

== system przyklad_mateusz/Subsystem1/Subsystem/enkoder/Triggered Subsystem ==
  In1 : Inport
  Trigger : TriggerPort  VariantControl=(inherit)
  Subtract : Sum  Inputs=+-
  Unit Delay : UnitDelay  SampleTime=-1  HasFrameUpgradeWarning=on
  Out1 : Outport
  wires:
  In1/1 -> Subtract/1, Unit Delay/1
  Unit Delay/1 -> Subtract/2
  Subtract/1 -> Out1/1

== system przyklad_mateusz/Subsystem1/Subsystem/kierunek obrotow/kierunek obrotów ==
  u : Inport
  Compare To Zero : simulink/Logic and Bit Operations/Compare To Zero  relop=>  OutDataTypeStr=boolean
  Logical Operator : Logic  Operator=NOT  AllPortsSameDT=off  OutDataTypeStr=boolean
  y : Outport
  Out2 : Outport  Port=2
  wires:
  Compare To Zero/1 -> y/1, Logical Operator/1
  Logical Operator/1 -> Out2/1
  u/1 -> Compare To Zero/1

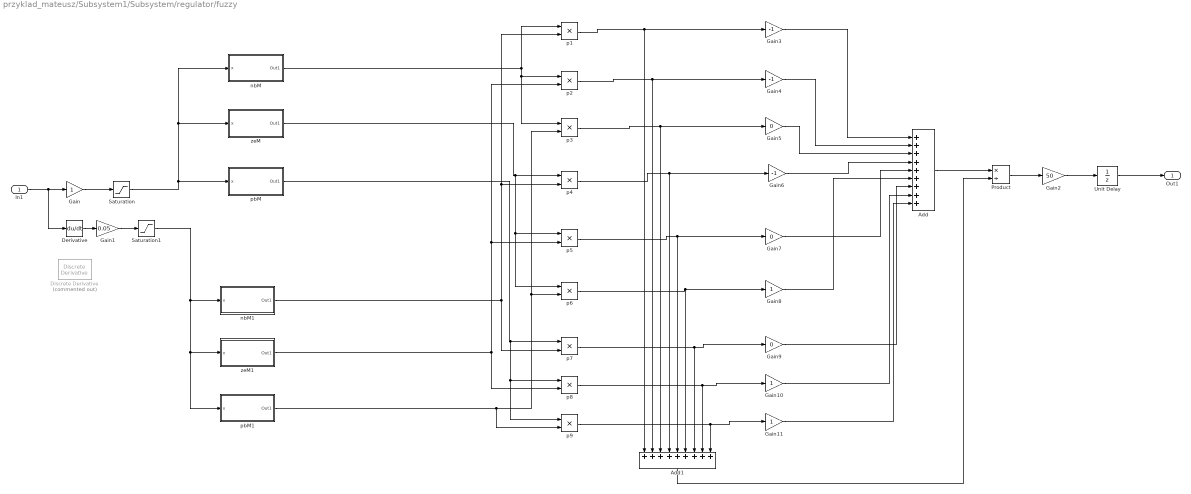
== system przyklad_mateusz/Subsystem1/Subsystem/regulator/fuzzy ==
  In1 : Inport
  Add : Sum  Inputs=+++++++++
  Add1 : Sum  Inputs=+++++++++
  Derivative : Derivative
  Discrete Derivative : simulink/Discrete/Discrete Derivative  Commented=on  gainval=1.0  ICPrevScaledInput=0.0  OutMin=[]  OutMax=[]  OutDataType=fixdt(1, 16)  OutScaling=2^-10  DoSatur=off
  Gain{,8,10..11} (4 alike) : Gain
  Gain1 : Gain  Gain=0.05
  Gain2 : Gain  Gain=50
  Gain3 : Gain  Gain=-1
  Gain4 : Gain  Gain=-1
  Gain5 : Gain  Gain=0
  Gain6 : Gain  Gain=-1
  Gain7 : Gain  Gain=0
  Gain9 : Gain  Gain=0
  Product : Product  Inputs=*/
  Saturation : Saturate  UpperLimit=1  LowerLimit=-1
  Saturation1 : Saturate  UpperLimit=1  LowerLimit=-1
  Unit Delay : UnitDelay  SampleTime=-1  HasFrameUpgradeWarning=on
  nbM : Subsystem
  nbM1 : Subsystem
  p{1..9} (9 alike) : Product
  pbM : Subsystem
  pbM1 : Subsystem
  zeM : Subsystem
  zeM1 : Subsystem
  Out1 : Outport
  wires:
  In1/1 -> Derivative/1, Gain/1
  Gain/1 -> Saturation/1
  Derivative/1 -> Gain1/1
  Gain1/1 -> Saturation1/1
  Gain2/1 -> Unit Delay/1
  Product/1 -> Gain2/1
  Saturation/1 -> zeM/1(x), nbM/1(x), pbM/1(x)
  Saturation1/1 -> nbM1/1(x), zeM1/1(x), pbM1/1(x)
  p1/1 -> Add1/1, Gain3/1
  p3/1 -> Gain5/1, Add1/3
  p2/1 -> Gain4/1, Add1/2
  p4/1 -> Gain6/1, Add1/4
  p5/1 -> Gain7/1, Add1/5
  p6/1 -> Gain8/1, Add1/6
  p7/1 -> Gain9/1, Add1/7
  p8/1 -> Gain10/1, Add1/8
  p9/1 -> Gain11/1, Add1/9
  nbM/1(Out1) -> p3/1, p2/1, p1/1
  nbM1/1(Out1) -> p7/2, p4/2, p1/2
  zeM1/1(Out1) -> p8/2, p5/2, p2/2
  pbM1/1(Out1) -> p9/2, p6/2, p3/2
  zeM/1(Out1) -> p6/1, p5/1, p4/1
  pbM/1(Out1) -> p9/1, p8/1, p7/1
  Gain3/1 -> Add/1
  Gain4/1 -> Add/2
  Gain5/1 -> Add/3
  Gain6/1 -> Add/4
  Gain7/1 -> Add/5
  Gain8/1 -> Add/6
  Gain9/1 -> Add/7
  Gain10/1 -> Add/8
  Gain11/1 -> Add/9
  Add/1 -> Product/1
  Add1/1 -> Product/2
  Unit Delay/1 -> Out1/1

== system przyklad_mateusz/obiekt/fuzzy/Fuzzy Logic Controller/__InputSSForSFun__ ==
  in : Inport
  __UniqueOutportName__1__ : Outport
  wires:
  in/1 -> __UniqueOutportName__1__/1

== system przyklad_mateusz/obiekt/fuzzy/Fuzzy Logic Controller/__OutputSSForSFun__ ==
  __UniqueInportName__1__ : Inport
  out : Outport  VectorParamsAs1DForOutWhenUnconnected=off
  wires:
  __UniqueInportName__1__/1 -> out/1  "defuzzifiedOutputs"

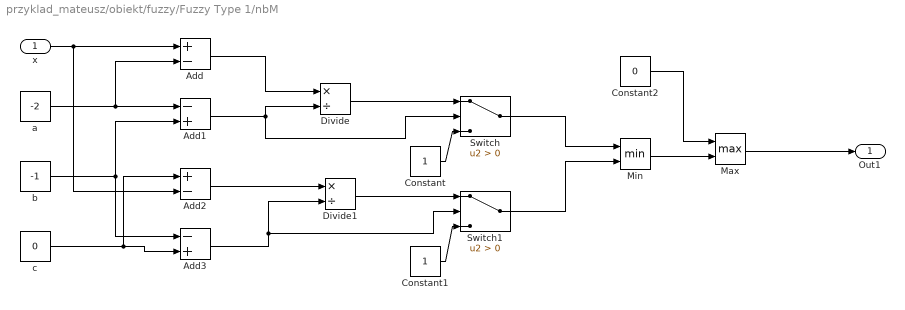
== system przyklad_mateusz/obiekt/fuzzy/Fuzzy Type 1/nbM ==
  x : Inport
  Add : Sum  Inputs=+-
  Add1 : Sum  Inputs=-+
  Add2 : Sum  Inputs=+-
  Add3 : Sum  Inputs=-+
  Constant : Constant
  Constant1 : Constant
  Constant2 : Constant  Value=0
  Divide : Product  Inputs=*/
  Divide1 : Product  Inputs=*/
  Max : MinMax  Function=max  Inputs=2
  Min : MinMax  Inputs=2
  Switch : Switch  Criteria=u2 > Threshold  SaturateOnIntegerOverflow=off  InputSameDT=off
  Switch1 : Switch  Criteria=u2 > Threshold  SaturateOnIntegerOverflow=off  InputSameDT=off
  a : Constant  Value=-2
  b : Constant  Value=-1
  c : Constant  Value=0
  Out1 : Outport
  wires:
  x/1 -> Add2/2, Add/1
  a/1 -> Add1/1, Add/2
  b/1 -> Add1/2, Add3/1
  c/1 -> Add2/1, Add3/2
  Add/1 -> Divide/1
  Divide1/1 -> Switch1/1
  Divide/1 -> Switch/1
  Add1/1 -> Switch/2, Divide/2
  Add2/1 -> Divide1/1
  Add3/1 -> Switch1/2, Divide1/2
  Constant/1 -> Switch/3
  Constant1/1 -> Switch1/3
  Switch/1 -> Min/1
  Switch1/1 -> Min/2
  Min/1 -> Max/2
  Constant2/1 -> Max/1
  Max/1 -> Out1/1

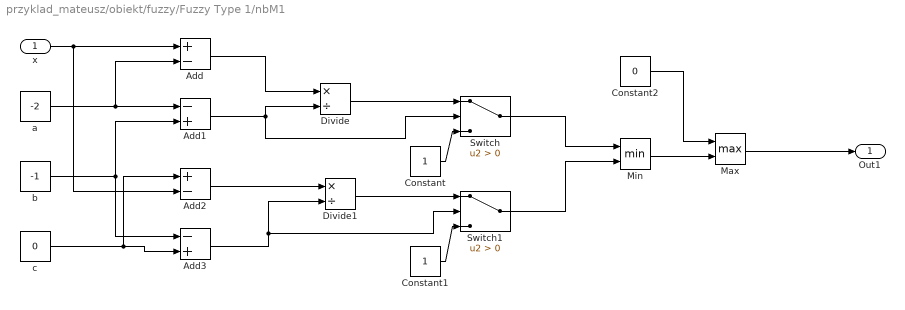
== system przyklad_mateusz/obiekt/fuzzy/Fuzzy Type 1/nbM1 ==
  x : Inport
  Add : Sum  Inputs=+-
  Add1 : Sum  Inputs=-+
  Add2 : Sum  Inputs=+-
  Add3 : Sum  Inputs=-+
  Constant : Constant
  Constant1 : Constant
  Constant2 : Constant  Value=0
  Divide : Product  Inputs=*/
  Divide1 : Product  Inputs=*/
  Max : MinMax  Function=max  Inputs=2
  Min : MinMax  Inputs=2
  Switch : Switch  Criteria=u2 > Threshold  SaturateOnIntegerOverflow=off  InputSameDT=off
  Switch1 : Switch  Criteria=u2 > Threshold  SaturateOnIntegerOverflow=off  InputSameDT=off
  a : Constant  Value=-2
  b : Constant  Value=-1
  c : Constant  Value=0
  Out1 : Outport
  wires:
  x/1 -> Add2/2, Add/1
  a/1 -> Add1/1, Add/2
  b/1 -> Add1/2, Add3/1
  c/1 -> Add2/1, Add3/2
  Add/1 -> Divide/1
  Divide1/1 -> Switch1/1
  Divide/1 -> Switch/1
  Add1/1 -> Switch/2, Divide/2
  Add2/1 -> Divide1/1
  Add3/1 -> Switch1/2, Divide1/2
  Constant/1 -> Switch/3
  Constant1/1 -> Switch1/3
  Switch/1 -> Min/1
  Switch1/1 -> Min/2
  Min/1 -> Max/2
  Constant2/1 -> Max/1
  Max/1 -> Out1/1

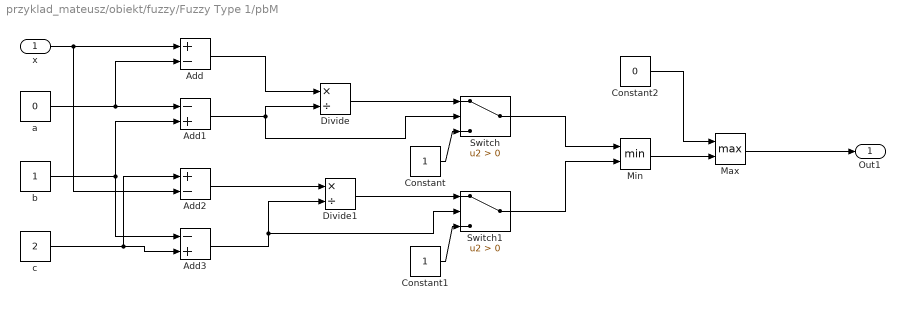
== system przyklad_mateusz/obiekt/fuzzy/Fuzzy Type 1/pbM ==
  x : Inport
  Add : Sum  Inputs=+-
  Add1 : Sum  Inputs=-+
  Add2 : Sum  Inputs=+-
  Add3 : Sum  Inputs=-+
  Constant : Constant
  Constant1 : Constant
  Constant2 : Constant  Value=0
  Divide : Product  Inputs=*/
  Divide1 : Product  Inputs=*/
  Max : MinMax  Function=max  Inputs=2
  Min : MinMax  Inputs=2
  Switch : Switch  Criteria=u2 > Threshold  SaturateOnIntegerOverflow=off  InputSameDT=off
  Switch1 : Switch  Criteria=u2 > Threshold  SaturateOnIntegerOverflow=off  InputSameDT=off
  a : Constant  Value=0
  b : Constant
  c : Constant  Value=2
  Out1 : Outport
  wires:
  x/1 -> Add2/2, Add/1
  a/1 -> Add1/1, Add/2
  b/1 -> Add1/2, Add3/1
  c/1 -> Add2/1, Add3/2
  Add/1 -> Divide/1
  Divide1/1 -> Switch1/1
  Divide/1 -> Switch/1
  Add1/1 -> Switch/2, Divide/2
  Add2/1 -> Divide1/1
  Add3/1 -> Switch1/2, Divide1/2
  Constant/1 -> Switch/3
  Constant1/1 -> Switch1/3
  Switch/1 -> Min/1
  Switch1/1 -> Min/2
  Min/1 -> Max/2
  Constant2/1 -> Max/1
  Max/1 -> Out1/1

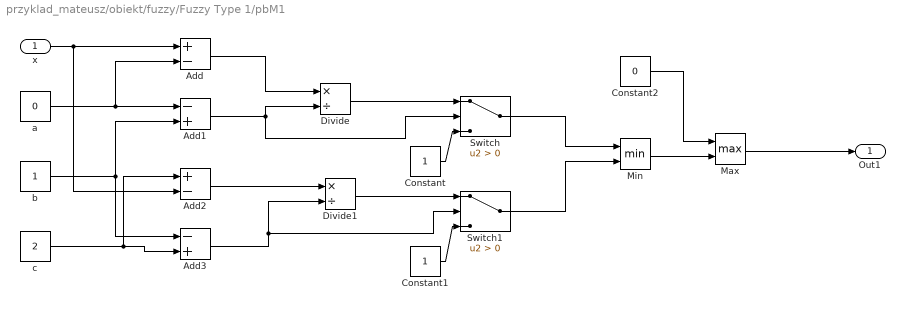
== system przyklad_mateusz/obiekt/fuzzy/Fuzzy Type 1/pbM1 ==
  x : Inport
  Add : Sum  Inputs=+-
  Add1 : Sum  Inputs=-+
  Add2 : Sum  Inputs=+-
  Add3 : Sum  Inputs=-+
  Constant : Constant
  Constant1 : Constant
  Constant2 : Constant  Value=0
  Divide : Product  Inputs=*/
  Divide1 : Product  Inputs=*/
  Max : MinMax  Function=max  Inputs=2
  Min : MinMax  Inputs=2
  Switch : Switch  Criteria=u2 > Threshold  SaturateOnIntegerOverflow=off  InputSameDT=off
  Switch1 : Switch  Criteria=u2 > Threshold  SaturateOnIntegerOverflow=off  InputSameDT=off
  a : Constant  Value=0
  b : Constant
  c : Constant  Value=2
  Out1 : Outport
  wires:
  x/1 -> Add2/2, Add/1
  a/1 -> Add1/1, Add/2
  b/1 -> Add1/2, Add3/1
  c/1 -> Add2/1, Add3/2
  Add/1 -> Divide/1
  Divide1/1 -> Switch1/1
  Divide/1 -> Switch/1
  Add1/1 -> Switch/2, Divide/2
  Add2/1 -> Divide1/1
  Add3/1 -> Switch1/2, Divide1/2
  Constant/1 -> Switch/3
  Constant1/1 -> Switch1/3
  Switch/1 -> Min/1
  Switch1/1 -> Min/2
  Min/1 -> Max/2
  Constant2/1 -> Max/1
  Max/1 -> Out1/1

== system przyklad_mateusz/obiekt/fuzzy/Fuzzy Type 1/zeM ==
  x : Inport
  Add : Sum  Inputs=+-
  Add1 : Sum  Inputs=-+
  Add2 : Sum  Inputs=+-
  Add3 : Sum  Inputs=-+
  Constant : Constant
  Constant1 : Constant
  Constant2 : Constant  Value=0
  Divide : Product  Inputs=*/
  Divide1 : Product  Inputs=*/
  Max : MinMax  Function=max  Inputs=2
  Min : MinMax  Inputs=2
  Switch : Switch  Criteria=u2 > Threshold  SaturateOnIntegerOverflow=off  InputSameDT=off
  Switch1 : Switch  Criteria=u2 > Threshold  SaturateOnIntegerOverflow=off  InputSameDT=off
  a : Constant  Value=-1
  b : Constant  Value=0
  c : Constant
  Out1 : Outport
  wires:
  x/1 -> Add2/2, Add/1
  a/1 -> Add1/1, Add/2
  b/1 -> Add1/2, Add3/1
  c/1 -> Add2/1, Add3/2
  Add/1 -> Divide/1
  Divide1/1 -> Switch1/1
  Divide/1 -> Switch/1
  Add1/1 -> Switch/2, Divide/2
  Add2/1 -> Divide1/1
  Add3/1 -> Switch1/2, Divide1/2
  Constant/1 -> Switch/3
  Constant1/1 -> Switch1/3
  Switch/1 -> Min/1
  Switch1/1 -> Min/2
  Min/1 -> Max/2
  Constant2/1 -> Max/1
  Max/1 -> Out1/1

== system przyklad_mateusz/obiekt/fuzzy/Fuzzy Type 1/zeM1 ==
  x : Inport
  Add : Sum  Inputs=+-
  Add1 : Sum  Inputs=-+
  Add2 : Sum  Inputs=+-
  Add3 : Sum  Inputs=-+
  Constant : Constant
  Constant1 : Constant
  Constant2 : Constant  Value=0
  Divide : Product  Inputs=*/
  Divide1 : Product  Inputs=*/
  Max : MinMax  Function=max  Inputs=2
  Min : MinMax  Inputs=2
  Switch : Switch  Criteria=u2 > Threshold  SaturateOnIntegerOverflow=off  InputSameDT=off
  Switch1 : Switch  Criteria=u2 > Threshold  SaturateOnIntegerOverflow=off  InputSameDT=off
  a : Constant  Value=-1
  b : Constant  Value=0
  c : Constant
  Out1 : Outport
  wires:
  x/1 -> Add2/2, Add/1
  a/1 -> Add1/1, Add/2
  b/1 -> Add1/2, Add3/1
  c/1 -> Add2/1, Add3/2
  Add/1 -> Divide/1
  Divide1/1 -> Switch1/1
  Divide/1 -> Switch/1
  Add1/1 -> Switch/2, Divide/2
  Add2/1 -> Divide1/1
  Add3/1 -> Switch1/2, Divide1/2
  Constant/1 -> Switch/3
  Constant1/1 -> Switch1/3
  Switch/1 -> Min/1
  Switch1/1 -> Min/2
  Min/1 -> Max/2
  Constant2/1 -> Max/1
  Max/1 -> Out1/1

== system przyklad_mateusz/obiekt/fuzzy/Fuzzy Type 2/nbM2 ==
  x : Inport
  Add : Sum  Inputs=+-
  Add1 : Sum  Inputs=-+
  Add2 : Sum  Inputs=+-
  Add3 : Sum  Inputs=-+
  Constant : Constant
  Constant1 : Constant
  Constant2 : Constant  Value=0
  Divide : Product  Inputs=*/
  Divide1 : Product  Inputs=*/
  Max : MinMax  Function=max  Inputs=2
  Min : MinMax  Inputs=2
  Switch : Switch  Criteria=u2 > Threshold  SaturateOnIntegerOverflow=off  InputSameDT=off
  Switch1 : Switch  Criteria=u2 > Threshold  SaturateOnIntegerOverflow=off  InputSameDT=off
  a : Constant  Value=-2
  b : Constant  Value=-1
  c : Constant  Value=0
  Out1 : Outport
  wires:
  Max/1 -> Out1/1
  Constant2/1 -> Max/1
  Min/1 -> Max/2
  Switch1/1 -> Min/2
  Switch/1 -> Min/1
  Constant1/1 -> Switch1/3
  Constant/1 -> Switch/3
  Add3/1 -> Divide1/2, Switch1/2
  Add2/1 -> Divide1/1
  Add1/1 -> Divide/2, Switch/2
  Divide/1 -> Switch/1
  Divide1/1 -> Switch1/1
  Add/1 -> Divide/1
  c/1 -> Add3/2, Add2/1
  b/1 -> Add3/1, Add1/2
  a/1 -> Add/2, Add1/1
  x/1 -> Add/1, Add2/2

== system przyklad_mateusz/obiekt/fuzzy/Fuzzy Type 2/nbM3 ==
  x : Inport
  Add : Sum  Inputs=+-
  Add1 : Sum  Inputs=-+
  Add2 : Sum  Inputs=+-
  Add3 : Sum  Inputs=-+
  Constant : Constant
  Constant1 : Constant
  Constant2 : Constant  Value=0
  Divide : Product  Inputs=*/
  Divide1 : Product  Inputs=*/
  Max : MinMax  Function=max  Inputs=2
  Min : MinMax  Inputs=2
  Switch : Switch  Criteria=u2 > Threshold  SaturateOnIntegerOverflow=off  InputSameDT=off
  Switch1 : Switch  Criteria=u2 > Threshold  SaturateOnIntegerOverflow=off  InputSameDT=off
  a : Constant  Value=-2
  b : Constant  Value=-1
  c : Constant  Value=0
  Out1 : Outport
  wires:
  Max/1 -> Out1/1
  Constant2/1 -> Max/1
  Min/1 -> Max/2
  Switch1/1 -> Min/2
  Switch/1 -> Min/1
  Constant1/1 -> Switch1/3
  Constant/1 -> Switch/3
  Add3/1 -> Divide1/2, Switch1/2
  Add2/1 -> Divide1/1
  Add1/1 -> Divide/2, Switch/2
  Divide/1 -> Switch/1
  Divide1/1 -> Switch1/1
  Add/1 -> Divide/1
  c/1 -> Add3/2, Add2/1
  b/1 -> Add3/1, Add1/2
  a/1 -> Add/2, Add1/1
  x/1 -> Add/1, Add2/2

== system przyklad_mateusz/obiekt/fuzzy/Fuzzy Type 2/nbM4 ==
  x : Inport
  Add : Sum  Inputs=+-
  Add1 : Sum  Inputs=-+
  Add2 : Sum  Inputs=+-
  Add3 : Sum  Inputs=-+
  Constant : Constant
  Constant1 : Constant
  Constant2 : Constant  Value=0
  Divide : Product  Inputs=*/
  Divide1 : Product  Inputs=*/
  Max : MinMax  Function=max  Inputs=2
  Min : MinMax  Inputs=2
  Switch : Switch  Criteria=u2 > Threshold  SaturateOnIntegerOverflow=off  InputSameDT=off
  Switch1 : Switch  Criteria=u2 > Threshold  SaturateOnIntegerOverflow=off  InputSameDT=off
  a : Constant  Value=-1.8
  b : Constant  Value=-1
  c : Constant  Value=-0.2
  Out1 : Outport
  wires:
  x/1 -> Add2/2, Add/1
  a/1 -> Add1/1, Add/2
  b/1 -> Add1/2, Add3/1
  c/1 -> Add2/1, Add3/2
  Add/1 -> Divide/1
  Divide1/1 -> Switch1/1
  Divide/1 -> Switch/1
  Add1/1 -> Switch/2, Divide/2
  Add2/1 -> Divide1/1
  Add3/1 -> Switch1/2, Divide1/2
  Constant/1 -> Switch/3
  Constant1/1 -> Switch1/3
  Switch/1 -> Min/1
  Switch1/1 -> Min/2
  Min/1 -> Max/2
  Constant2/1 -> Max/1
  Max/1 -> Out1/1
